simulink model "gm_lorenz_model"  (R2018a)
settings: Solver=FixedStepAuto  StartTime=0.0  StopTime=inf  RelTol=1e-3  EnableMultiTasking=on
libraries: simulink x7, simulink_extras x1
settings Model: Creator=labuser  LastModifiedBy=labuser
settings SolverCC: PositivePriorityOrder=on  AutoInsertRateTranBlk=on
settings OptimizationCC: BlockReduction=off  ConditionallyExecuteInputs=off  DefaultParameterBehavior=Inlined  EnhancedBackFolding=on  PassReuseOutputArgsThreshold=0  MaxStackSize=64  OptimizeBlockOrder=speed  DifferentSizesBufferReuse=on  OptimizationCustomize=off
settings DebuggingCC: AlgebraicLoopMsg=error  InheritedTsInSrcMsg=none  ParameterTunabilityLossMsg=error
settings HardwareCC: ProdBitPerPointer=32  ProdBitPerSizeT=32  ProdBitPerPtrDiffT=32  ProdLargestAtomicFloat=None  ProdIntDivRoundTo=Undefined  ProdEndianess=Unspecified  ProdWordSize=32  ProdHWDeviceType=ASIC/FPGA->ASIC/FPGA  TargetBitPerPointer=64  TargetBitPerSizeT=64  TargetBitPerPtrDiffT=64  TargetLongLongMode=on  TargetIntDivRoundTo=Zero  TargetEndianess=LittleEndian  TargetWordSize=64  TargetHWDeviceType=Custom Processor->MATLAB Host Computer  ProdEqTarget=off
settings SFSimCC: MATLABDynamicMemAlloc=off
settings RTWCC: Description=Generic Real-Time Target  GenerateReport=on  Toolchain=ARM Development Studio Altera Edition (DS-5 AE)  LaunchReport=on
settings CodeAppCC: ForceParamTrailComments=on  OperatorAnnotations=on
settings GRTTargetCC: TargetLangStandard=C89/C90 (ANSI)

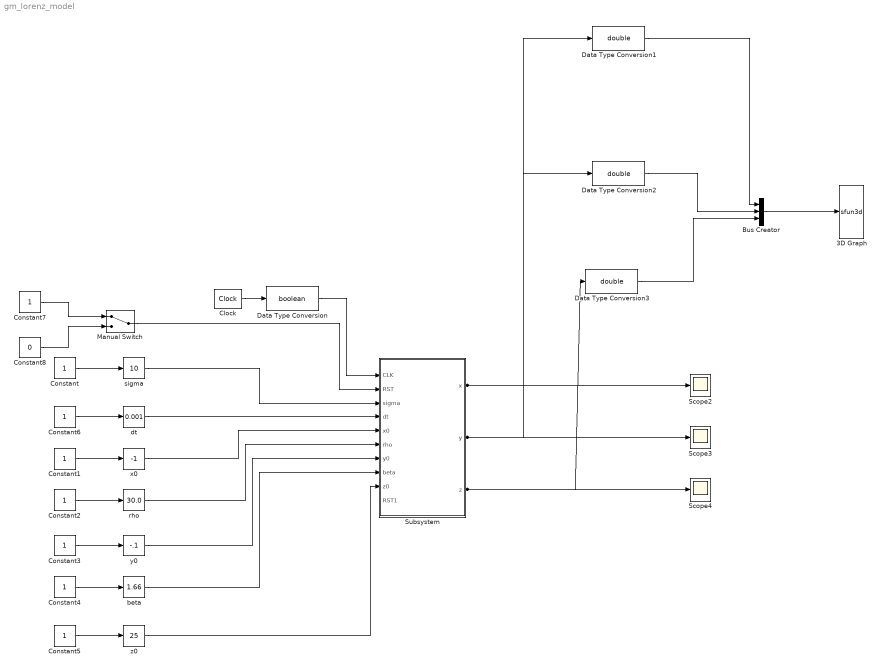
== system gm_lorenz_model ==
  3D Graph : S-Function  LoadFcn=if exist('sfun3d','file'), sfun3d([],[],[],'LoadBlock'); end  FunctionName=sfun3d  Parameters=ax,T,np,cp,gd,ls,mk,mx,hd,tb  SFunctionDeploymentMode=off  EnableBusSupport=off  mask(3D Graph){np=1, ax=[-30 30 -30 30 0 50], mx=2000, T=0.01, cp=[370 -234 -207], gd=on, hd=on, tb=off, ls=-, mk=none}
      mask prompts: np "Number of moving points (lines)"; ax "Range: [xmin xmax  ymin ymax zmin zmax]"; mx "Max number of points in each line"; T "Sampling Time"; cp "Camera position (use [0 0 1] for 2D XY view)"; gd "Grid (on|off)"; hd "HeadMarkers (on|off)"; tb "Toolbar (on|off)"; ls "LineStyle"; mk "LineMarker"
      mask help:
      | This block plots the position of several points in the XYZ space. The input contains the coordinates of all the points (x1,y1,z1,x2,y2,z2,...).
      | The number of moving points (lines), the XYZ ranges, sampling time, camera position, and grid (among other things) can be set as mask parameters.
      settings: CopyFcn=if exist('sfun3d','file'), sfun3d([],[],[],'CopyBlock'); end  DeleteFcn=if exist('sfun3d','file'), sfun3d([],[],[],'DeleteBlock'); end  NameChangeFcn=if exist('sfun3d','file'), sfun3d([],[],[],'NameChange'); end
      mask Help:
      | This block plots the position of several points in the XYZ space. The input contains the coordinates of all the points (x1,y1,z1,x2,y2,z2,...).
      | The number of moving points (lines), the XYZ ranges, sampling time, camera position, and grid (among other things) can be set as mask parameters.
      mask TypeOptions ls: - | -- | : | -. | none
      mask TypeOptions mk: none | . | + | o | * | x | square | diamond | v | ^ | > | < | pentagram | hexagram
      mask Display: plot([.05 .95 .95 .05 .05],[.45 .45 .95 .95 .45], 0.5+cos(0:0.1:2*pi)*0.3,0.7+sin(0:0.1:2*pi)*0.2)
  Bus Creator : BusCreator  Inputs=3
  Clock : simulink_extras/Flip Flops/Clock  period=0.001
  Constant{,1..6} (7 alike) : Constant  OutDataTypeStr=fixdt(1,27,20)  SampleTime=-1
  Constant7 : Constant  OutDataTypeStr=boolean  SampleTime=-1
  Constant8 : Constant  Value=0  OutDataTypeStr=boolean  SampleTime=-1
  Data Type Conversion : DataTypeConversion  OutDataTypeStr=boolean
  Data Type Conversion1 : DataTypeConversion  OutDataTypeStr=double
  Data Type Conversion2 : DataTypeConversion  OutDataTypeStr=double
  Data Type Conversion3 : DataTypeConversion  OutDataTypeStr=double
  Manual Switch : ManualSwitch
  Scope2 : Scope
  Scope3 : Scope
  Scope4 : Scope
  Subsystem : Subsystem  TreatAsAtomicUnit=on
  beta : simulink/Math Operations/Slider Gain  gain=1.66  low=0  high=5
  dt : simulink/Math Operations/Slider Gain  gain=0.001  low=0  high=100
  rho : simulink/Math Operations/Slider Gain  gain=30.0  low=0  high=50
  sigma : simulink/Math Operations/Slider Gain  gain=10  low=-20  high=20
  x0 : simulink/Math Operations/Slider Gain  gain=-1  low=-2  high=2
  y0 : simulink/Math Operations/Slider Gain  gain=-.1  low=-1  high=1
  z0 : simulink/Math Operations/Slider Gain  gain=25  low=0  high=50
  wires:
  Subsystem/2(y) -> Data Type Conversion2/1, Scope3/1
  Subsystem/3(z) -> Data Type Conversion3/1, Scope4/1
  Subsystem/1(x) -> Scope2/1, Data Type Conversion1/1
  beta/1 -> Subsystem/8(beta)
  z0/1 -> Subsystem/9(z0)
  y0/1 -> Subsystem/7(y0)
  rho/1 -> Subsystem/6(rho)
  x0/1 -> Subsystem/5(x0)
  dt/1 -> Subsystem/4(dt)
  Constant/1 -> sigma/1
  Constant4/1 -> beta/1
  Constant6/1 -> dt/1
  Constant3/1 -> y0/1
  Constant5/1 -> z0/1
  Constant2/1 -> rho/1
  Constant1/1 -> x0/1
  sigma/1 -> Subsystem/3(sigma)
  Data Type Conversion3/1 -> Bus Creator/3
  Data Type Conversion2/1 -> Bus Creator/2
  Data Type Conversion1/1 -> Bus Creator/1
  Bus Creator/1 -> 3D Graph/1
  Data Type Conversion/1 -> Subsystem/1(CLK)
  Clock/1 -> Data Type Conversion/1
  Manual Switch/1 -> Subsystem/2(RST)
  Constant8/1 -> Manual Switch/2
  Constant7/1 -> Manual Switch/1

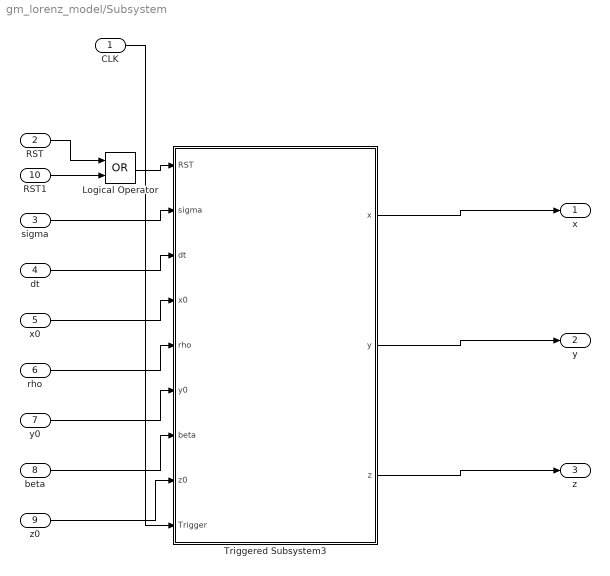
== system gm_lorenz_model/Subsystem ==
  CLK : Inport  OutDataTypeStr=boolean  PortDimensions=1  SampleTime=0.0005
  RST : Inport  Port=2  OutDataTypeStr=boolean  PortDimensions=1  SampleTime=0.0005
  sigma : Inport  Port=3  OutDataTypeStr=fixdt(1, 27, 20)  PortDimensions=1  SampleTime=0.0005
  dt : Inport  Port=4  OutDataTypeStr=fixdt(1, 27, 20)  PortDimensions=1  SampleTime=0.0005
  x0 : Inport  Port=5  OutDataTypeStr=fixdt(1, 27, 20)  PortDimensions=1  SampleTime=0.0005
  rho : Inport  Port=6  OutDataTypeStr=fixdt(1, 27, 20)  PortDimensions=1  SampleTime=0.0005
  y0 : Inport  Port=7  OutDataTypeStr=fixdt(1, 27, 20)  PortDimensions=1  SampleTime=0.0005
  beta : Inport  Port=8  OutDataTypeStr=fixdt(1, 27, 20)  PortDimensions=1  SampleTime=0.0005
  z0 : Inport  Port=9  OutDataTypeStr=fixdt(1, 27, 20)  PortDimensions=1  SampleTime=0.0005
  RST1 : Inport  Port=10  OutDataTypeStr=boolean  PortDimensions=1
  Logical Operator : Logic  Operator=OR  AllPortsSameDT=off  OutDataTypeStr=boolean
  Triggered Subsystem3 : Subsystem
  x : Outport  OutDataTypeStr=fixdt(1,27,20)
  y : Outport  Port=2  OutDataTypeStr=fixdt(1,27,20)
  z : Outport  Port=3  OutDataTypeStr=fixdt(1,27,20)
  wires:
  CLK/1 -> Triggered Subsystem3/9(Trigger)
  RST/1 -> Logical Operator/1
  sigma/1 -> Triggered Subsystem3/2(sigma)
  dt/1 -> Triggered Subsystem3/3(dt)
  x0/1 -> Triggered Subsystem3/4(x0)
  rho/1 -> Triggered Subsystem3/5(rho)
  y0/1 -> Triggered Subsystem3/6(y0)
  beta/1 -> Triggered Subsystem3/7(beta)
  z0/1 -> Triggered Subsystem3/8(z0)
  RST1/1 -> Logical Operator/2
  Logical Operator/1 -> Triggered Subsystem3/1(RST)
  Triggered Subsystem3/1(x) -> x/1
  Triggered Subsystem3/2(y) -> y/1
  Triggered Subsystem3/3(z) -> z/1

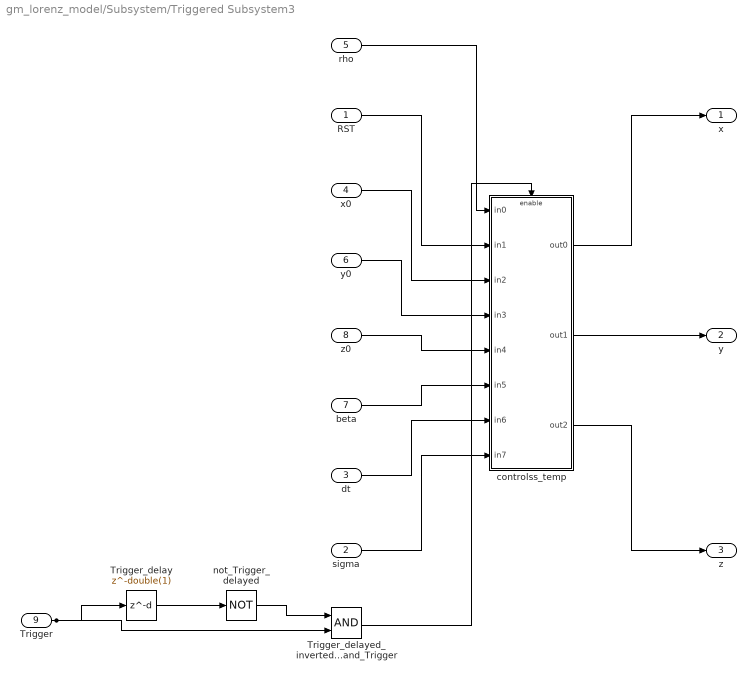
== system gm_lorenz_model/Subsystem/Triggered Subsystem3 ==
  RST : Inport  OutDataTypeStr=boolean  PortDimensions=1  SampleTime=0.0005
  sigma : Inport  Port=2  OutDataTypeStr=fixdt(1,27,20)  PortDimensions=1  SampleTime=0.0005
  dt : Inport  Port=3  OutDataTypeStr=fixdt(1,27,20)  PortDimensions=1  SampleTime=0.0005
  x0 : Inport  Port=4  OutDataTypeStr=fixdt(1,27,20)  PortDimensions=1  SampleTime=0.0005
  rho : Inport  Port=5  OutDataTypeStr=fixdt(1,27,20)  PortDimensions=1  SampleTime=0.0005
  y0 : Inport  Port=6  OutDataTypeStr=fixdt(1,27,20)  PortDimensions=1  SampleTime=0.0005
  beta : Inport  Port=7  OutDataTypeStr=fixdt(1,27,20)  PortDimensions=1  SampleTime=0.0005
  z0 : Inport  Port=8  OutDataTypeStr=fixdt(1,27,20)  PortDimensions=1  SampleTime=0.0005
  Trigger : Inport  Port=9  OutDataTypeStr=boolean  SampleTime=0.0005
  Trigger_delay : Delay  DelayLength=double(1)  InitialCondition=1  InputProcessing=Inherited
  Trigger_delayed_inverted_and_Trigger : Logic  AllPortsSameDT=off  OutDataTypeStr=boolean  SampleTime=0.0005
  controlss_temp : Subsystem
  not_Trigger_delayed : Logic  Operator=NOT  Inputs=1  AllPortsSameDT=off  OutDataTypeStr=boolean  SampleTime=0.0005
  x : Outport  OutDataTypeStr=fixdt(1,27,20)  InitialOutput=0
  y : Outport  Port=2  OutDataTypeStr=fixdt(1,27,20)  InitialOutput=0
  z : Outport  Port=3  OutDataTypeStr=fixdt(1,27,20)  InitialOutput=0
  wires:
  Trigger/1 -> Trigger_delayed_inverted_and_Trigger/2, Trigger_delay/1
  RST/1 -> controlss_temp/2(in1)
  sigma/1 -> controlss_temp/8(in7)
  dt/1 -> controlss_temp/7(in6)
  x0/1 -> controlss_temp/3(in2)
  rho/1 -> controlss_temp/1(in0)
  y0/1 -> controlss_temp/4(in3)
  beta/1 -> controlss_temp/6(in5)
  z0/1 -> controlss_temp/5(in4)
  controlss_temp/1(out0) -> x/1
  controlss_temp/2(out1) -> y/1
  controlss_temp/3(out2) -> z/1
  Trigger_delay/1 -> not_Trigger_delayed/1
  not_Trigger_delayed/1 -> Trigger_delayed_inverted_and_Trigger/1
  Trigger_delayed_inverted_and_Trigger/1 -> controlss_temp/Enable

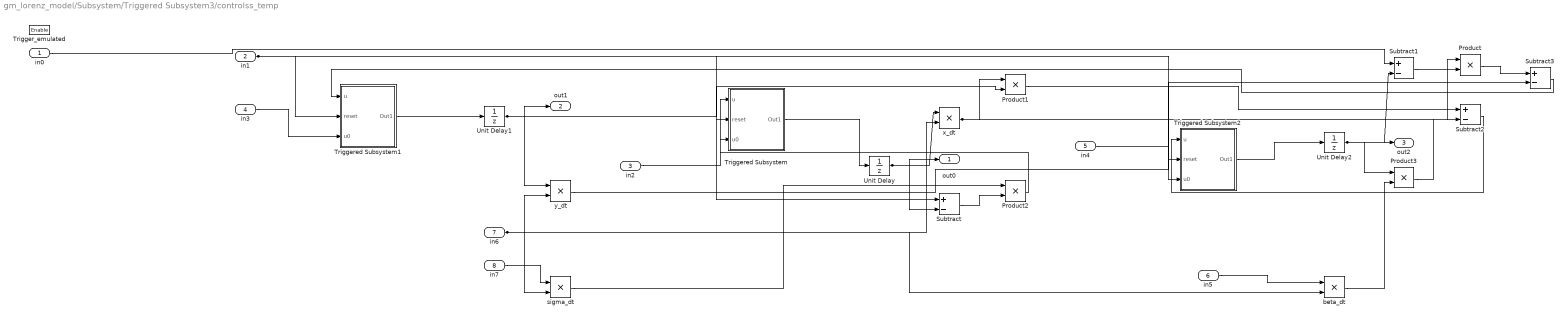
== system gm_lorenz_model/Subsystem/Triggered Subsystem3/controlss_temp ==
  in0 : Inport  OutDataTypeStr=fixdt(1, 27, 20)  SampleTime=0.0005
  in1 : Inport  Port=2  OutDataTypeStr=boolean  SampleTime=0.0005
  in2 : Inport  Port=3  OutDataTypeStr=fixdt(1, 27, 20)  SampleTime=0.0005
  in3 : Inport  Port=4  OutDataTypeStr=fixdt(1, 27, 20)  SampleTime=0.0005
  in4 : Inport  Port=5  OutDataTypeStr=fixdt(1, 27, 20)  SampleTime=0.0005
  in5 : Inport  Port=6  OutDataTypeStr=fixdt(1, 27, 20)  SampleTime=0.0005
  in6 : Inport  Port=7  OutDataTypeStr=fixdt(1, 27, 20)  SampleTime=0.0005
  in7 : Inport  Port=8  OutDataTypeStr=fixdt(1, 27, 20)  SampleTime=0.0005
  Trigger_emulated : EnablePort  OutDataTypeStr=boolean
  Product{,1..3} (4 alike) : Product  Inputs=**  OutDataTypeStr=fixdt(1, 27, 20)  SampleTime=0.0005
  Subtract{,1..3} (4 alike) : Sum  Inputs=+-  AccumDataTypeStr=fixdt(1, 27, 20)  OutDataTypeStr=fixdt(1, 27, 20)  SampleTime=0.0005
  Triggered Subsystem : Subsystem
  Triggered Subsystem1 : Subsystem
  Triggered Subsystem2 : Subsystem
  Unit Delay : UnitDelay  InitialCondition=fi(0,1,27,20,'hex','0000000')  SampleTime=0.0005
  Unit Delay1 : UnitDelay  InitialCondition=fi(0,1,27,20,'hex','0000000')  SampleTime=0.0005
  Unit Delay2 : UnitDelay  InitialCondition=fi(0,1,27,20,'hex','0000000')  SampleTime=0.0005
  beta_dt : Product  Inputs=**  OutDataTypeStr=fixdt(1, 27, 20)  SampleTime=0.0005
  sigma_dt : Product  Inputs=**  OutDataTypeStr=fixdt(1, 27, 20)  SampleTime=0.0005
  x_dt : Product  Inputs=**  OutDataTypeStr=fixdt(1, 27, 20)  SampleTime=0.0005
  y_dt : Product  Inputs=**  OutDataTypeStr=fixdt(1, 27, 20)  SampleTime=0.0005
  out0 : Outport  OutDataTypeStr=fixdt(1, 27, 20)  InitialOutput=0
  out1 : Outport  Port=2  OutDataTypeStr=fixdt(1, 27, 20)  InitialOutput=0
  out2 : Outport  Port=3  OutDataTypeStr=fixdt(1, 27, 20)  InitialOutput=0
  wires:
  Product/1 -> Subtract3/1
  Product1/1 -> Subtract2/1
  Product2/1 -> Triggered Subsystem/1(u)
  Product3/1 -> Subtract2/2
  Subtract/1 -> Product2/2
  Subtract1/1 -> Product/2
  Subtract2/1 -> Triggered Subsystem2/1(u)
  Subtract3/1 -> Triggered Subsystem1/1(u)
  Triggered Subsystem/1(Out1) -> Unit Delay/1
  Triggered Subsystem1/1(Out1) -> Unit Delay1/1
  Triggered Subsystem2/1(Out1) -> Unit Delay2/1
  beta_dt/1 -> Product3/2
  sigma_dt/1 -> Product2/1
  x_dt/1 -> Product1/1, Product/1
  y_dt/1 -> Subtract3/2
  Unit Delay/1 -> x_dt/1, Subtract/2, out0/1
  Unit Delay1/1 -> y_dt/1, Subtract/1, Product1/2, out1/1
  Unit Delay2/1 -> Subtract1/2, Product3/1, out2/1
  in0/1 -> Subtract1/1
  in1/1 -> Triggered Subsystem/2(reset), Triggered Subsystem1/2(reset), Triggered Subsystem2/2(reset)
  in2/1 -> Triggered Subsystem/3(u0)
  in3/1 -> Triggered Subsystem1/3(u0)
  in4/1 -> Triggered Subsystem2/3(u0)
  in5/1 -> beta_dt/1
  in6/1 -> y_dt/2, x_dt/2, sigma_dt/2, beta_dt/2
  in7/1 -> sigma_dt/1

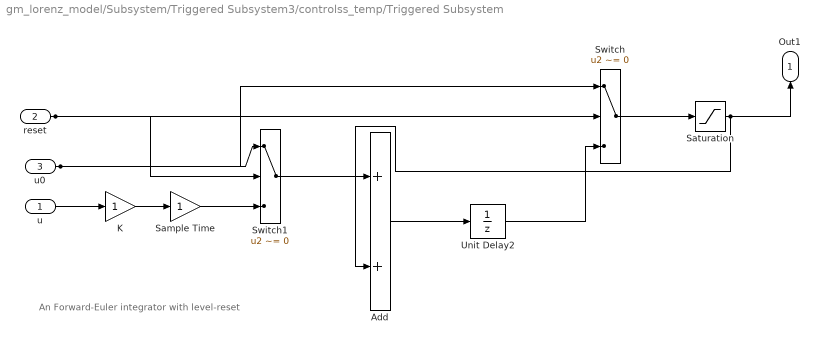
== system gm_lorenz_model/Subsystem/Triggered Subsystem3/controlss_temp/Triggered Subsystem ==
  note: An Forward-Euler integrator with level-reset
  u : Inport  PortDimensions=1  SampleTime=0.0005
  reset : Inport  Port=2  PortDimensions=1  SampleTime=0.0005
  u0 : Inport  Port=3  PortDimensions=1  SampleTime=0.0005
  Add : Sum
  K : Gain  OutDataTypeStr=Inherit: Same as input
  Sample Time : Gain  OutDataTypeStr=Inherit: Same as input
  Saturation : Saturate  UpperLimit=63  LowerLimit=-63
  Switch : Switch  Criteria=u2 ~= 0  OutDataTypeStr=Inherit: Inherit via back propagation
  Switch1 : Switch  Criteria=u2 ~= 0  OutDataTypeStr=Inherit: Inherit via back propagation
  Unit Delay2 : UnitDelay  SampleTime=-1
  Out1 : Outport  InitialOutput=0
  wires:
  u/1 -> K/1
  reset/1 -> Switch1/2, Switch/2
  u0/1 -> Switch1/1, Switch/1
  Add/1 -> Unit Delay2/1
  K/1 -> Sample Time/1
  Sample Time/1 -> Switch1/3
  Saturation/1 -> Add/2, Out1/1
  Switch/1 -> Saturation/1
  Switch1/1 -> Add/1
  Unit Delay2/1 -> Switch/3

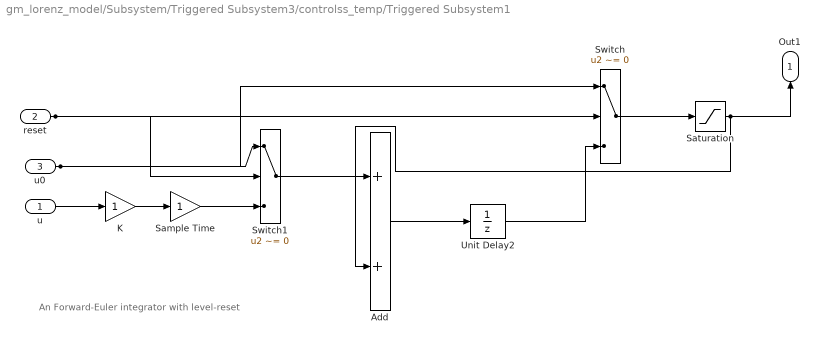
== system gm_lorenz_model/Subsystem/Triggered Subsystem3/controlss_temp/Triggered Subsystem1 ==
  note: An Forward-Euler integrator with level-reset
  u : Inport  PortDimensions=1  SampleTime=0.0005
  reset : Inport  Port=2  PortDimensions=1  SampleTime=0.0005
  u0 : Inport  Port=3  PortDimensions=1  SampleTime=0.0005
  Add : Sum
  K : Gain  OutDataTypeStr=Inherit: Same as input
  Sample Time : Gain  OutDataTypeStr=Inherit: Same as input
  Saturation : Saturate  UpperLimit=63  LowerLimit=-63
  Switch : Switch  Criteria=u2 ~= 0  OutDataTypeStr=Inherit: Inherit via back propagation
  Switch1 : Switch  Criteria=u2 ~= 0  OutDataTypeStr=Inherit: Inherit via back propagation
  Unit Delay2 : UnitDelay  SampleTime=-1
  Out1 : Outport  InitialOutput=0
  wires:
  Unit Delay2/1 -> Switch/3
  Switch1/1 -> Add/1
  Switch/1 -> Saturation/1
  Saturation/1 -> Out1/1, Add/2
  Sample Time/1 -> Switch1/3
  K/1 -> Sample Time/1
  Add/1 -> Unit Delay2/1
  u0/1 -> Switch/1, Switch1/1
  reset/1 -> Switch/2, Switch1/2
  u/1 -> K/1

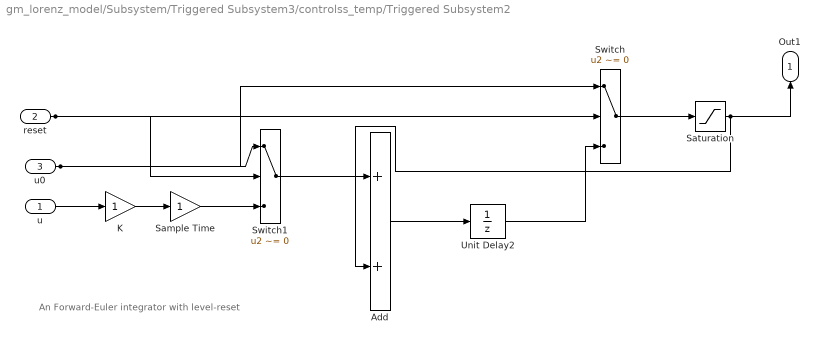
== system gm_lorenz_model/Subsystem/Triggered Subsystem3/controlss_temp/Triggered Subsystem2 ==
  note: An Forward-Euler integrator with level-reset
  u : Inport  PortDimensions=1  SampleTime=0.0005
  reset : Inport  Port=2  PortDimensions=1  SampleTime=0.0005
  u0 : Inport  Port=3  PortDimensions=1  SampleTime=0.0005
  Add : Sum
  K : Gain  OutDataTypeStr=Inherit: Same as input
  Sample Time : Gain  OutDataTypeStr=Inherit: Same as input
  Saturation : Saturate  UpperLimit=63  LowerLimit=-63
  Switch : Switch  Criteria=u2 ~= 0  OutDataTypeStr=Inherit: Inherit via back propagation
  Switch1 : Switch  Criteria=u2 ~= 0  OutDataTypeStr=Inherit: Inherit via back propagation
  Unit Delay2 : UnitDelay  SampleTime=-1
  Out1 : Outport  InitialOutput=0
  wires:
  Unit Delay2/1 -> Switch/3
  Switch1/1 -> Add/1
  Switch/1 -> Saturation/1
  Saturation/1 -> Out1/1, Add/2
  Sample Time/1 -> Switch1/3
  K/1 -> Sample Time/1
  Add/1 -> Unit Delay2/1
  u0/1 -> Switch/1, Switch1/1
  reset/1 -> Switch/2, Switch1/2
  u/1 -> K/1
